simulink model "ventilator"  (R2020a)
settings: Solver=VariableStepAuto  StartTime=0.0  StopTime=20  FixedStep=0.001  MaxStep=0.01  RelTol=1e-3  AbsTol=1e-3
InitFcn:
  | load('params');
  | 
  | Transport_Delay = 0.001; % s
  | 
  | Zephyr_FS = 50; % SLPM
  | HSC_FS = 160; % mbar
  | 
  | P_supply =1; % bar
  | 
  | T_room = 20; % degC
  | RH_room = 0.1;
  | T_humidifier = 40; % degC
  | T_body = 37; % degC
  | 
  | L_tube = 1; % m
  | D_tube = 0.022; % m
  | L_trachea = 0.15; % m
  | D_trachea = 0.015; % m
  | 
  | Chamber_volume = 0.2; % L
  | FRC = 2; % L
  | 
  | % Conversion factors
  | cmH2O_to_Pa = 98.0665;
  | L_to_m3 = 1e-3;
undefined symbols (not defined in the file or in its folder): zephyr
libraries: fl_lib x101, nesl_utility x26
(part 2 of 2)

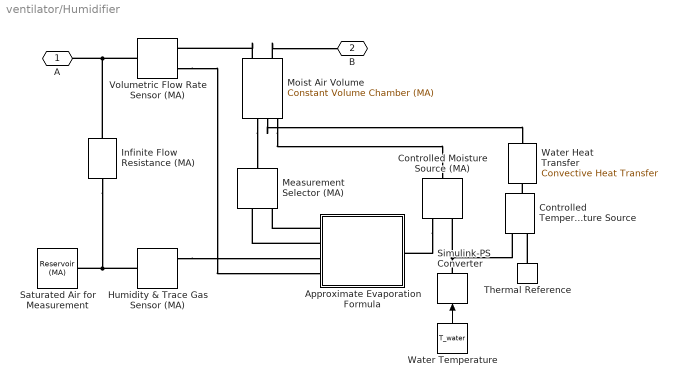
== system ventilator/Humidifier ==
  Approximate Evaporation Formula : Subsystem
  Controlled Temperature Source : fl_lib/Thermal/Thermal Sources/Controlled Temperature Source
      settings: SourceProductBaseCode=MT,SS
  Controlled Moisture Source (MA) : fl_lib/Moist Air/Sources/Moisture & Trace Gas Sources/Controlled Moisture Source (MA)  moisture_source_spec=foundation.enum.moisture_source_spec.vapor
      settings: SourceProductBaseCode=MT,SS  InternalSimscapePortConfiguration="{\"Bottom\":[],\"Left\":[{\"id\":\"S\",\"label\":\"S\",\"type\":\"foundation.moist_air.moist_air_source\"}],\"Right\":[{\"id\":\"M\",\"label\":\"M\",\"type\":\"input\"},{\"id\":\"T\",\"label\":\"T\",\"type\":\"input\"}],\"Top\":[]}"
  Humidity & Trace Gas Sensor (MA) : fl_lib/Moist Air/Sensors/Humidity & Trace Gas Sensor (MA)  moisture_spec=foundation.enum.moisture_spec.mole_fraction  trace_gas_spec=foundation.enum.trace_gas_spec.mass_fraction
      settings: SourceProductBaseCode=MT,SS  InternalSimscapePortConfiguration="{\"Bottom\":[],\"Left\":[{\"id\":\"A\",\"label\":\"A\",\"type\":\"foundation.moist_air.moist_air\"}],\"Right\":[{\"id\":\"W\",\"label\":\"W\",\"type\":\"output\"},{\"id\":\"G\",\"label\":\"G\",\"type\":\"output\"}],\"Top\":[]}"
  Infinite Flow Resistance (MA) : fl_lib/Moist Air/Elements/Infinite Flow Resistance (MA)  p_specify=off  p_priority=None  p=0 MPa  p_nominal_specify=off  p_nominal_unit=MPa  p_nominal_value=1  T_specify=off  T_priority=None  T=0 K  T_nominal_specify=off  T_nominal_unit=K  T_nominal_value=1  x_w_specify=off  x_w_priority=None  x_w=0  x_w_nominal_specify=off  x_w_nominal_unit=1  x_w_nominal_value=1  x_g_specify=off  x_g_priority=None  x_g=0  x_g_nominal_specify=off  x_g_nominal_unit=1  x_g_nominal_value=1
      settings: SourceProductBaseCode=MT,SS  InternalSimscapePortConfiguration="{\"Bottom\":[],\"Left\":[{\"id\":\"A\",\"label\":\"A\",\"type\":\"foundation.moist_air.moist_air\"}],\"Right\":[{\"id\":\"B\",\"label\":\"B\",\"type\":\"foundation.moist_air.moist_air\"}],\"Top\":[]}"
  Measurement Selector (MA) : fl_lib/Moist Air/Sensors/Measurement Selector (MA)  moisture_spec=foundation.enum.moisture_spec.mole_fraction  trace_gas_spec=foundation.enum.trace_gas_spec.mass_fraction
      settings: SourceProductBaseCode=MT,SS
  Moist Air Volume : fl_lib/Moist Air/Elements/Constant Volume Chamber (MA)  volume=V_humidifier m^3  num_ports=foundation.enum.num_ports.two  area_A=pi*D_tube^2/4 m^2  area_B=pi*D_tube^2/4 m^2  area_C=0.01 m^2  area_D=0.01 m^2  RH_ws=1  time_constant=1e-3 s  moisture_trace_gas_source=foundation.enum.moisture_trace_gas_source.controlled  moisture_source_spec=foundation.enum.moisture_source_spec.vapor  moisture_mass_flow=0 kg/s  moisture_temperature_spec=foundation.enum.temperature_spec.atmospheric  moisture_temperature=293.15 K  trace_gas_mass_flow=0 kg/s  trace_gas_temperature_spec=foundation.enum.temperature_spec.atmospheric  trace_gas_temperature=293.15 K  p_I_specify=off  p_I_priority=High  p_I=0.101325 MPa  p_I_nominal_specify=off  p_I_nominal_unit=MPa  p_I_nominal_value=1  T_I_specify=on  T_I_priority=High  T_I=T_room degC  T_I_nominal_specify=off  T_I_nominal_unit=K  T_I_nominal_value=1  RH_I_specify=on  RH_I_priority=High  RH_I=RH_room  RH_I_nominal_specify=off  RH_I_nominal_unit=1  RH_I_nominal_value=1  x_w_I_specify=off  x_w_I_priority=None  x_w_I=0  x_w_I_nominal_specify=off  x_w_I_nominal_unit=1  x_w_I_nominal_value=1  y_w_I_specify=off  y_w_I_priority=None  y_w_I=0  y_w_I_nominal_specify=off  y_w_I_nominal_unit=1  y_w_I_nominal_value=1  HR_I_specify=off  HR_I_priority=None  HR_I=0  HR_I_nominal_specify=off  HR_I_nominal_unit=1  HR_I_nominal_value=1  x_g_I_specify=off  x_g_I_priority=High  x_g_I=0  x_g_I_nominal_specify=off  x_g_I_nominal_unit=1  x_g_I_nominal_value=1  y_g_I_specify=off  y_g_I_priority=None  y_g_I=0  y_g_I_nominal_specify=off  y_g_I_nominal_unit=1  y_g_I_nominal_value=1
      settings: SourceProductBaseCode=MT,SS  InternalSimscapePortConfiguration="{\"Bottom\":[],\"Left\":[{\"id\":\"A\",\"label\":\"A\",\"type\":\"foundation.moist_air.moist_air\"},{\"id\":\"B\",\"label\":\"B\",\"type\":\"foundation.moist_air.moist_air\"}],\"Right\":[{\"id\":\"W\",\"label\":\"W\",\"type\":\"output\"},{\"id\":\"F\",\"label\":\"F\",\"type\":\"output\"},{\"id\":\"H\",\"label\":\"H\",\"type\":\"foundation.thermal.thermal\"},{\"id\":\"S\",\"label\":\"S\",\"type\":\"foundation.moist_air.moist_air_source\"}],\"Top\":[]}"
  Saturated Air for Measurement : fl_lib/Moist Air/Elements/Reservoir (MA)  pressure_spec=1  reservoir_pressure=0.101325 MPa  temperature_spec=2  reservoir_temperature=T_water degC  moisture_spec=1  reservoir_RH=1  reservoir_x_w=0.01  reservoir_y_w=0.01  reservoir_HR=0.01  trace_gas_spec=1  reservoir_x_g=0  reservoir_y_g=0.001  RH_ws=1  area_A=A_humidifier m^2
      settings: SourceProductBaseCode=MT,SS
  Simulink-PS Converter : nesl_utility/Simulink-PS Converter  PhysicalDomain=network_engine_domain  SubClassName=ps_input  LeftPortType=input  RightPortType=output  PseudoPeriodic=off  Frequencies=[]  NoiseDistribution=none  NoiseParameters=[]  Unit=degC  AffineConversion=on  FilteringAndDerivatives=provide  SimscapeFilterOrder=1  InputFilterTimeConstant=0.001  UdotUserProvided=0
      settings: SourceProductBaseCode=MT,SS
  Thermal Reference : fl_lib/Thermal/Thermal Elements/Thermal Reference
      settings: SourceProductBaseCode=MT,SS
  Volumetric Flow Rate Sensor (MA) : fl_lib/Moist Air/Sensors/Volumetric Flow Rate Sensor (MA)  volumetric_flow_conditions=foundation.enum.volumetric_flow_conditions.actual  p_std=0.101325 MPa  T_std=20 degC  RH_std=0.65
      settings: SourceProductBaseCode=MT,SS  InternalSimscapePortConfiguration="{\"Bottom\":[],\"Left\":[{\"id\":\"A\",\"label\":\"A\",\"type\":\"foundation.moist_air.moist_air\"}],\"Right\":[{\"id\":\"B\",\"label\":\"B\",\"type\":\"foundation.moist_air.moist_air\"},{\"id\":\"V\",\"label\":\"V\",\"type\":\"output\"}],\"Top\":[]}"
  Water Temperature : Constant  Value=T_water
  Water Heat Transfer : fl_lib/Thermal/Thermal Elements/Convective Heat Transfer  area=A_humidifier m^2  heat_tr_coeff=20 W/(m^2 * K)  T_specify=off  T_priority=None  T=0 K  T_nominal_specify=off  T_nominal_unit=K  T_nominal_value=1  Q_specify=off  Q_priority=None  Q=0 W  Q_nominal_specify=off  Q_nominal_unit=W  Q_nominal_value=1
      settings: SourceProductBaseCode=MT,SS
  A : PMIOPort  Side=Left
  B : PMIOPort  Port=2  Side=Right
  wires:
  Water Temperature/1 -> Simulink-PS Converter/1
  connections:
  Volumetric Flow Rate Sensor (MA)/LConn1 -- A/RConn1 -- Infinite Flow Resistance (MA)/RConn1
  Moist Air Volume/LConn1 -- Volumetric Flow Rate Sensor (MA)/RConn1
  Moist Air Volume/LConn2 -- B/RConn1
  Humidity & Trace Gas Sensor (MA)/RConn1 -- Approximate Evaporation Formula/LConn3
  Volumetric Flow Rate Sensor (MA)/RConn2 -- Approximate Evaporation Formula/LConn4
  Controlled Moisture Source (MA)/RConn1 -- Approximate Evaporation Formula/RConn1
  Moist Air Volume/RConn4 -- Controlled Moisture Source (MA)/LConn1
  Moist Air Volume/RConn2 -- Measurement Selector (MA)/LConn1
  Infinite Flow Resistance (MA)/LConn1 -- Saturated Air for Measurement/LConn1 -- Humidity & Trace Gas Sensor (MA)/LConn1
  Controlled Temperature Source/LConn1 -- Water Heat Transfer/RConn1
  Simulink-PS Converter/RConn1 -- Controlled Temperature Source/RConn1 -- Controlled Moisture Source (MA)/RConn2
  Moist Air Volume/RConn3 -- Water Heat Transfer/LConn1
  Thermal Reference/LConn1 -- Controlled Temperature Source/RConn2
  Approximate Evaporation Formula/LConn1 -- Measurement Selector (MA)/RConn1
  Approximate Evaporation Formula/LConn2 -- Measurement Selector (MA)/RConn3

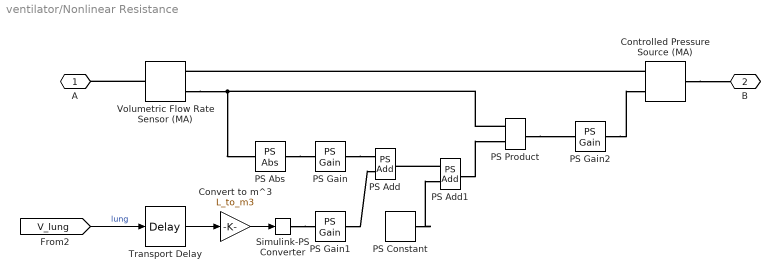
== system ventilator/Nonlinear Resistance ==
  Controlled Pressure Source (MA) : fl_lib/Moist Air/Sources/Controlled Pressure Source (MA)  power_spec=foundation.enum.power_spec.isentropic  area_A=pi*D_trachea^2/4 m^2  area_B=pi*D_trachea^2/4 m^2
      settings: SourceProductBaseCode=SS  InternalSimscapePortConfiguration="{\"Bottom\":[],\"Left\":[{\"id\":\"A\",\"label\":\"A\",\"type\":\"foundation.moist_air.moist_air\"},{\"id\":\"P\",\"label\":\"P\",\"type\":\"input\"}],\"Right\":[{\"id\":\"B\",\"label\":\"B\",\"type\":\"foundation.moist_air.moist_air\"}],\"Top\":[]}"
  Convert to m^3 : Gain  Gain=L_to_m3
  PS Abs : fl_lib/Physical Signals/Nonlinear Operators/PS Abs
      settings: SourceProductBaseCode=SS  InternalSimscapePortConfiguration="{\"Bottom\":[],\"Left\":[{\"id\":\"I\",\"label\":\"\",\"type\":\"input\"}],\"Right\":[{\"id\":\"O\",\"label\":\"\",\"type\":\"output\"}],\"Top\":[]}"
  PS Add : fl_lib/Physical Signals/Functions/PS Add
  PS Add1 : fl_lib/Physical Signals/Functions/PS Add
  PS Constant : fl_lib/Physical Signals/Sources/PS Constant  constant=R0 * 1e3 / 1e-3 Pa * s / m^3
  PS Gain : fl_lib/Physical Signals/Functions/PS Gain  gain=Kf * 1e3 / 1e-6 Pa * s^2 / m^6
  PS Gain1 : fl_lib/Physical Signals/Functions/PS Gain  gain=Kv * 1e3 / 1e-6 Pa * s / m^6
  PS Gain2 : fl_lib/Physical Signals/Functions/PS Gain  gain=-1
  PS Product : fl_lib/Physical Signals/Functions/PS Product
  Simulink-PS Converter : nesl_utility/Simulink-PS Converter  PhysicalDomain=network_engine_domain  SubClassName=ps_input  LeftPortType=input  RightPortType=output  PseudoPeriodic=off  Frequencies=[]  NoiseDistribution=none  NoiseParameters=[]  Unit=m^3  AffineConversion=off  FilteringAndDerivatives=provide  SimscapeFilterOrder=1  InputFilterTimeConstant=0.001  UdotUserProvided=0
  Transport Delay : TransportDelay  DelayTime=Transport_Delay  BufferSize=2048
  Volumetric Flow Rate Sensor (MA) : fl_lib/Moist Air/Sensors/Volumetric Flow Rate Sensor (MA)  volumetric_flow_conditions=foundation.enum.volumetric_flow_conditions.actual  p_std=0.101325 MPa  T_std=20 degC  RH_std=0.65
      settings: SourceProductBaseCode=SS  InternalSimscapePortConfiguration="{\"Bottom\":[],\"Left\":[{\"id\":\"A\",\"label\":\"A\",\"type\":\"foundation.moist_air.moist_air\"}],\"Right\":[{\"id\":\"B\",\"label\":\"B\",\"type\":\"foundation.moist_air.moist_air\"},{\"id\":\"V\",\"label\":\"V\",\"type\":\"output\"}],\"Top\":[]}"
  A : PMIOPort  Side=Left
  B : PMIOPort  Port=2  Side=Right
  wires:
  [V_lung] -> Transport Delay/1  "lung"
  Convert to m^3/1 -> Simulink-PS Converter/1
  Transport Delay/1 -> Convert to m^3/1
  connections:
  Volumetric Flow Rate Sensor (MA)/RConn2 -- PS Abs/LConn1 -- PS Product/LConn1
  Volumetric Flow Rate Sensor (MA)/LConn1 -- A/RConn1
  PS Abs/RConn1 -- PS Gain/LConn1
  PS Gain/RConn1 -- PS Add/LConn1
  PS Add1/LConn1 -- PS Add/RConn1
  PS Constant/RConn1 -- PS Add1/LConn2
  PS Add1/RConn1 -- PS Product/LConn2
  Simulink-PS Converter/RConn1 -- PS Gain1/LConn1
  PS Gain1/RConn1 -- PS Add/LConn2
  Controlled Pressure Source (MA)/LConn1 -- Volumetric Flow Rate Sensor (MA)/RConn1
  Controlled Pressure Source (MA)/RConn1 -- B/RConn1
  PS Gain2/RConn1 -- Controlled Pressure Source (MA)/LConn2
  PS Product/RConn1 -- PS Gain2/LConn1

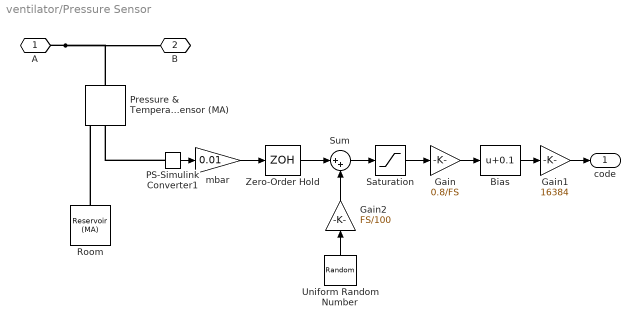
== system ventilator/Pressure Sensor ==
  Bias : Bias  Bias=0.1
  Gain : Gain  Gain=0.8/FS
  Gain1 : Gain  Gain=16384
  Gain2 : Gain  Gain=FS/100
  PS-Simulink Converter1 : nesl_utility/PS-Simulink Converter  PhysicalDomain=network_engine_domain  SubClassName=ps_output  LeftPortType=input  RightPortType=output  PseudoPeriodic=off  Frequencies=[]  Unit=inherit  AffineConversion=off
  Pressure & Temperature Sensor (MA) : fl_lib/Moist Air/Sensors/Pressure & Temperature Sensor (MA)
      settings: SourceProductBaseCode=MT,SS  InternalSimscapePortConfiguration="{\"Bottom\":[],\"Left\":[{\"id\":\"A\",\"label\":\"A\",\"type\":\"foundation.moist_air.moist_air\"}],\"Right\":[{\"id\":\"B\",\"label\":\"B\",\"type\":\"foundation.moist_air.moist_air\"},{\"id\":\"P\",\"label\":\"P\",\"type\":\"output\"},{\"id\":\"T\",\"label\":\"T\",\"type\":\"output\"}],\"Top\":[]}"
  Room : fl_lib/Moist Air/Elements/Reservoir (MA)  pressure_spec=foundation.enum.pressure_spec.atmospheric  reservoir_pressure=0.101325 MPa  temperature_spec=foundation.enum.temperature_spec.specified  reservoir_temperature=T_room degC  moisture_spec=foundation.enum.moisture_spec.relative_humidity  reservoir_RH=RH_room  reservoir_x_w=0.01  reservoir_y_w=0.01  reservoir_HR=0.01  trace_gas_spec=foundation.enum.trace_gas_spec.mass_fraction  reservoir_x_g=0  reservoir_y_g=0.001  RH_ws=1  area_A=pi*D_tube^2/4 m^2
      settings: SourceProductBaseCode=MT,SS
  Saturation : Saturate  UpperLimit=FS  LowerLimit=0
  Sum : Sum  Inputs=|++
  Uniform Random Number : UniformRandomNumber  SampleTime=Ts
  Zero-Order Hold : ZeroOrderHold  SampleTime=Ts
  mbar : Gain  Gain=0.01
  A : PMIOPort  Side=Left
  B : PMIOPort  Port=2  Side=Right
  code : Outport
  wires:
  Saturation/1 -> Gain/1
  Gain1/1 -> code/1
  Bias/1 -> Gain1/1
  Gain/1 -> Bias/1
  Sum/1 -> Saturation/1
  mbar/1 -> Zero-Order Hold/1
  Zero-Order Hold/1 -> Sum/1
  Uniform Random Number/1 -> Gain2/1
  Gain2/1 -> Sum/2
  PS-Simulink Converter1/1 -> mbar/1
  connections:
  PS-Simulink Converter1/LConn1 -- Pressure & Temperature Sensor (MA)/RConn2
  Room/LConn1 -- Pressure & Temperature Sensor (MA)/RConn1
  A/RConn1 -- B/RConn1 -- Pressure & Temperature Sensor (MA)/LConn1

== system ventilator/Proportional Inlet Valve ==
  duty_cycle : Inport
  Apply Actual Conditions : Subsystem
  Controlled Volumetric Flow Rate Source (MA) : fl_lib/Moist Air/Sources/Controlled Volumetric Flow Rate Source (MA)  power_spec=foundation.enum.power_spec.isentropic  volumetric_flow_conditions=foundation.enum.volumetric_flow_conditions.actual  p_std=0.101325 MPa  T_std=20 degC  RH_std=0.65  area_A=pi*D_tube^2/4 m^2  area_B=pi*D_tube^2/4 m^2
      settings: SourceProductBaseCode=SS  InternalSimscapePortConfiguration="{\"Bottom\":[],\"Left\":[{\"id\":\"A\",\"label\":\"A\",\"type\":\"foundation.moist_air.moist_air\"},{\"id\":\"V\",\"label\":\"V\",\"type\":\"input\"}],\"Right\":[{\"id\":\"B\",\"label\":\"B\",\"type\":\"foundation.moist_air.moist_air\"}],\"Top\":[]}"
  PS Constant : fl_lib/Physical Signals/Sources/PS Constant  constant=1e5 * valve.preload_offset Pa
  PS Lookup Table (2D) : fl_lib/Physical Signals/Lookup Tables/PS Lookup Table (2D)  x1=1e5 * valve.pressure Pa  x2=valve.duty_cycle  f=(1e-3/60) * valve.flow_rate m^3/s  interp_method=simscape.enum.interpolation.linear  extrap_method=simscape.enum.extrapolation.linear
      settings: SourceProductBaseCode=SS
  PS Subtract : fl_lib/Physical Signals/Functions/PS Subtract
  PS Transfer Function : fl_lib/Physical Signals/Linear Operators/PS Transfer Function  transfer_function_type=foundation.enum.transfer_function_type.lag  T=tau s  T1=2 s  T2=1 s  y0=0 m^3/s
      settings: SourceProductBaseCode=SS  InternalSimscapePortConfiguration="{\"Bottom\":[],\"Left\":[{\"id\":\"U\",\"label\":\"\",\"type\":\"input\"}],\"Right\":[{\"id\":\"Y\",\"label\":\"\",\"type\":\"output\"}],\"Top\":[]}"
  Pressure & Temperature Sensor (MA) : fl_lib/Moist Air/Sensors/Pressure & Temperature Sensor (MA)
      settings: SourceProductBaseCode=MT,SS  InternalSimscapePortConfiguration="{\"Bottom\":[],\"Left\":[{\"id\":\"A\",\"label\":\"A\",\"type\":\"foundation.moist_air.moist_air\"}],\"Right\":[{\"id\":\"B\",\"label\":\"B\",\"type\":\"foundation.moist_air.moist_air\"},{\"id\":\"P\",\"label\":\"P\",\"type\":\"output\"},{\"id\":\"T\",\"label\":\"T\",\"type\":\"output\"}],\"Top\":[]}"
  Saturation : Saturate  UpperLimit=100  LowerLimit=0
  Simulink-PS Converter : nesl_utility/Simulink-PS Converter  PhysicalDomain=network_engine_domain  SubClassName=ps_input  LeftPortType=input  RightPortType=output  PseudoPeriodic=off  Frequencies=[]  NoiseDistribution=none  NoiseParameters=[]  Unit=1  AffineConversion=off  FilteringAndDerivatives=provide  SimscapeFilterOrder=1  InputFilterTimeConstant=0.001  UdotUserProvided=0
  A : PMIOPort  Side=Left
  B : PMIOPort  Port=2  Side=Right
  wires:
  duty_cycle/1 -> Saturation/1
  Saturation/1 -> Simulink-PS Converter/1
  connections:
  Controlled Volumetric Flow Rate Source (MA)/LConn1 -- Pressure & Temperature Sensor (MA)/LConn1 -- A/RConn1
  Controlled Volumetric Flow Rate Source (MA)/RConn1 -- Pressure & Temperature Sensor (MA)/RConn1 -- B/RConn1
  PS Lookup Table (2D)/RConn1 -- Apply Actual Conditions/LConn1
  PS Transfer Function/RConn1 -- Controlled Volumetric Flow Rate Source (MA)/LConn2
  Apply Actual Conditions/RConn1 -- PS Transfer Function/LConn1
  PS Lookup Table (2D)/LConn2 -- Simulink-PS Converter/RConn1
  PS Subtract/LConn1 -- Pressure & Temperature Sensor (MA)/RConn2
  PS Subtract/RConn1 -- PS Lookup Table (2D)/LConn1
  PS Subtract/LConn2 -- PS Constant/RConn1

== system ventilator/Safety Vent Trap ==
  PS Transfer Function : fl_lib/Physical Signals/Linear Operators/PS Transfer Function  transfer_function_type=foundation.enum.transfer_function_type.lag  T=tau s  T1=2 s  T2=1 s  y0=1e-10 m^2
      settings: SourceProductBaseCode=SS  InternalSimscapePortConfiguration="{\"Bottom\":[],\"Left\":[{\"id\":\"U\",\"label\":\"\",\"type\":\"input\"}],\"Right\":[{\"id\":\"Y\",\"label\":\"\",\"type\":\"output\"}],\"Top\":[]}"
  Pressure & Temperature Sensor (MA) : fl_lib/Moist Air/Sensors/Pressure & Temperature Sensor (MA)
      settings: SourceProductBaseCode=MT,SS  InternalSimscapePortConfiguration="{\"Bottom\":[],\"Left\":[{\"id\":\"A\",\"label\":\"A\",\"type\":\"foundation.moist_air.moist_air\"}],\"Right\":[{\"id\":\"B\",\"label\":\"B\",\"type\":\"foundation.moist_air.moist_air\"},{\"id\":\"P\",\"label\":\"P\",\"type\":\"output\"},{\"id\":\"T\",\"label\":\"T\",\"type\":\"output\"}],\"Top\":[]}"
  Pressure to Area : fl_lib/Physical Signals/Lookup Tables/PS Lookup Table (1D)  x=[-0.2 -0.1 0 0.2 0.5 0.8 1 1.1 1.2]*(p_max - p_crack) + p_crack Pa  f=[0 0 0 0.2 0.5 0.8 1 1 1]*(pi*D_nozzle^2/4 - 1e-10) + 1e-10 m^2  interp_method=simscape.enum.interpolation.smooth  extrap_method=simscape.enum.extrapolation.nearest
      settings: SourceProductBaseCode=MT,SS
  Valve : fl_lib/Moist Air/Elements/Local Restriction (MA)  restriction_type=foundation.enum.restriction_type.variable  restriction_area=0.001 m^2  min_area=1e-10 m^2  max_area=pi*D_nozzle^2/4 m^2  area=pi*D_tube^2/4 m^2  Cd=0.8  B_lam=0.999
      settings: SourceProductBaseCode=MT,SS
  A : PMIOPort  Side=Left
  B : PMIOPort  Port=2  Side=Right
  connections:
  Pressure & Temperature Sensor (MA)/LConn1 -- Valve/LConn1 -- A/RConn1
  Pressure & Temperature Sensor (MA)/RConn1 -- Valve/RConn1 -- B/RConn1
  Pressure & Temperature Sensor (MA)/RConn2 -- Pressure to Area/LConn1
  PS Transfer Function/LConn1 -- Pressure to Area/RConn1
  PS Transfer Function/RConn1 -- Valve/LConn2

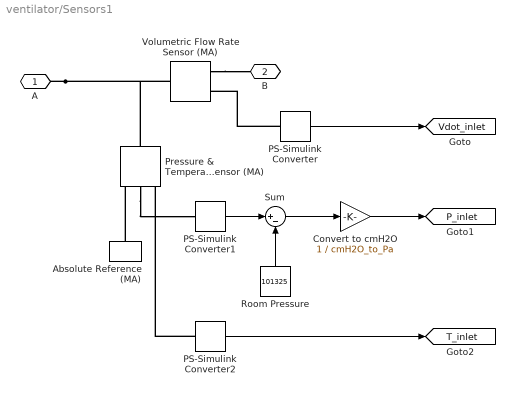
== system ventilator/Sensors1 ==
  Absolute Reference (MA) : fl_lib/Moist Air/Elements/Absolute Reference (MA)
      settings: SourceProductBaseCode=MT,SS
  Convert to cmH2O : Gain  Gain=1 / cmH2O_to_Pa
  PS-Simulink Converter : nesl_utility/PS-Simulink Converter  PhysicalDomain=network_engine_domain  SubClassName=ps_output  LeftPortType=input  RightPortType=output  PseudoPeriodic=off  Frequencies=[]  Unit=l/min  AffineConversion=off
      settings: SourceProductBaseCode=MT,SS
  PS-Simulink Converter1 : nesl_utility/PS-Simulink Converter  PhysicalDomain=network_engine_domain  SubClassName=ps_output  LeftPortType=input  RightPortType=output  PseudoPeriodic=off  Frequencies=[]  Unit=Pa  AffineConversion=off
      settings: SourceProductBaseCode=MT,SS
  PS-Simulink Converter2 : nesl_utility/PS-Simulink Converter  PhysicalDomain=network_engine_domain  SubClassName=ps_output  LeftPortType=input  RightPortType=output  PseudoPeriodic=off  Frequencies=[]  Unit=K  AffineConversion=off
      settings: SourceProductBaseCode=MT,SS
  Pressure & Temperature Sensor (MA) : fl_lib/Moist Air/Sensors/Pressure & Temperature Sensor (MA)
      settings: SourceProductBaseCode=MT,SS  InternalSimscapePortConfiguration="{\"Bottom\":[],\"Left\":[{\"id\":\"A\",\"label\":\"A\",\"type\":\"foundation.moist_air.moist_air\"}],\"Right\":[{\"id\":\"B\",\"label\":\"B\",\"type\":\"foundation.moist_air.moist_air\"},{\"id\":\"P\",\"label\":\"P\",\"type\":\"output\"},{\"id\":\"T\",\"label\":\"T\",\"type\":\"output\"}],\"Top\":[]}"
  Room Pressure : Constant  Value=101325
  Sum : Sum  Inputs=|+-
  Volumetric Flow Rate Sensor (MA) : fl_lib/Moist Air/Sensors/Volumetric Flow Rate Sensor (MA)  volumetric_flow_conditions=foundation.enum.volumetric_flow_conditions.actual  p_std=0.101325 MPa  T_std=20 degC  RH_std=0.65
      settings: SourceProductBaseCode=MT,SS  InternalSimscapePortConfiguration="{\"Bottom\":[],\"Left\":[{\"id\":\"A\",\"label\":\"A\",\"type\":\"foundation.moist_air.moist_air\"}],\"Right\":[{\"id\":\"B\",\"label\":\"B\",\"type\":\"foundation.moist_air.moist_air\"},{\"id\":\"V\",\"label\":\"V\",\"type\":\"output\"}],\"Top\":[]}"
  A : PMIOPort  Side=Left
  B : PMIOPort  Port=2  Side=Right
  tag scope: P_inlet=global, T_inlet=global, Vdot_inlet=global
  wires:
  Room Pressure/1 -> Sum/2
  Sum/1 -> Convert to cmH2O/1
  PS-Simulink Converter1/1 -> Sum/1
  Convert to cmH2O/1 -> [P_inlet]
  PS-Simulink Converter/1 -> [Vdot_inlet]
  PS-Simulink Converter2/1 -> [T_inlet]
  connections:
  Pressure & Temperature Sensor (MA)/RConn2 -- PS-Simulink Converter1/LConn1
  Absolute Reference (MA)/LConn1 -- Pressure & Temperature Sensor (MA)/RConn1
  Volumetric Flow Rate Sensor (MA)/RConn1 -- B/RConn1
  A/RConn1 -- Pressure & Temperature Sensor (MA)/LConn1 -- Volumetric Flow Rate Sensor (MA)/LConn1
  PS-Simulink Converter/LConn1 -- Volumetric Flow Rate Sensor (MA)/RConn2
  PS-Simulink Converter2/LConn1 -- Pressure & Temperature Sensor (MA)/RConn3

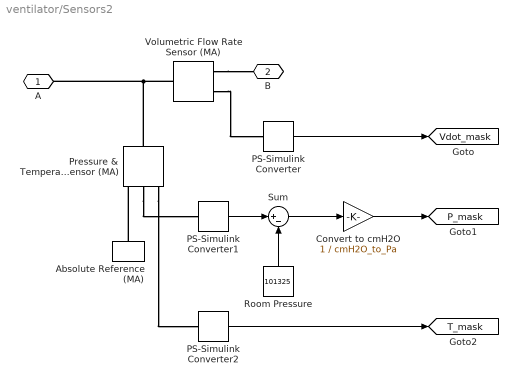
== system ventilator/Sensors2 ==
  Absolute Reference (MA) : fl_lib/Moist Air/Elements/Absolute Reference (MA)
      settings: SourceProductBaseCode=MT,SS
  Convert to cmH2O : Gain  Gain=1 / cmH2O_to_Pa
  PS-Simulink Converter : nesl_utility/PS-Simulink Converter  PhysicalDomain=network_engine_domain  SubClassName=ps_output  LeftPortType=input  RightPortType=output  PseudoPeriodic=off  Frequencies=[]  Unit=l/min  AffineConversion=off
      settings: SourceProductBaseCode=MT,SS
  PS-Simulink Converter1 : nesl_utility/PS-Simulink Converter  PhysicalDomain=network_engine_domain  SubClassName=ps_output  LeftPortType=input  RightPortType=output  PseudoPeriodic=off  Frequencies=[]  Unit=Pa  AffineConversion=off
      settings: SourceProductBaseCode=MT,SS
  PS-Simulink Converter2 : nesl_utility/PS-Simulink Converter  PhysicalDomain=network_engine_domain  SubClassName=ps_output  LeftPortType=input  RightPortType=output  PseudoPeriodic=off  Frequencies=[]  Unit=K  AffineConversion=off
      settings: SourceProductBaseCode=MT,SS
  Pressure & Temperature Sensor (MA) : fl_lib/Moist Air/Sensors/Pressure & Temperature Sensor (MA)
      settings: SourceProductBaseCode=MT,SS  InternalSimscapePortConfiguration="{\"Bottom\":[],\"Left\":[{\"id\":\"A\",\"label\":\"A\",\"type\":\"foundation.moist_air.moist_air\"}],\"Right\":[{\"id\":\"B\",\"label\":\"B\",\"type\":\"foundation.moist_air.moist_air\"},{\"id\":\"P\",\"label\":\"P\",\"type\":\"output\"},{\"id\":\"T\",\"label\":\"T\",\"type\":\"output\"}],\"Top\":[]}"
  Room Pressure : Constant  Value=101325
  Sum : Sum  Inputs=|+-
  Volumetric Flow Rate Sensor (MA) : fl_lib/Moist Air/Sensors/Volumetric Flow Rate Sensor (MA)  volumetric_flow_conditions=foundation.enum.volumetric_flow_conditions.actual  p_std=0.101325 MPa  T_std=20 degC  RH_std=0.65
      settings: SourceProductBaseCode=MT,SS  InternalSimscapePortConfiguration="{\"Bottom\":[],\"Left\":[{\"id\":\"A\",\"label\":\"A\",\"type\":\"foundation.moist_air.moist_air\"}],\"Right\":[{\"id\":\"B\",\"label\":\"B\",\"type\":\"foundation.moist_air.moist_air\"},{\"id\":\"V\",\"label\":\"V\",\"type\":\"output\"}],\"Top\":[]}"
  A : PMIOPort  Side=Left
  B : PMIOPort  Port=2  Side=Right
  tag scope: P_mask=global, T_mask=global, Vdot_mask=global
  wires:
  PS-Simulink Converter/1 -> [Vdot_mask]
  Convert to cmH2O/1 -> [P_mask]
  PS-Simulink Converter1/1 -> Sum/1
  Sum/1 -> Convert to cmH2O/1
  Room Pressure/1 -> Sum/2
  PS-Simulink Converter2/1 -> [T_mask]
  connections:
  Volumetric Flow Rate Sensor (MA)/LConn1 -- Pressure & Temperature Sensor (MA)/LConn1 -- A/RConn1
  Volumetric Flow Rate Sensor (MA)/RConn1 -- B/RConn1
  Volumetric Flow Rate Sensor (MA)/RConn2 -- PS-Simulink Converter/LConn1
  Absolute Reference (MA)/LConn1 -- Pressure & Temperature Sensor (MA)/RConn1
  Pressure & Temperature Sensor (MA)/RConn2 -- PS-Simulink Converter1/LConn1
  Pressure & Temperature Sensor (MA)/RConn3 -- PS-Simulink Converter2/LConn1

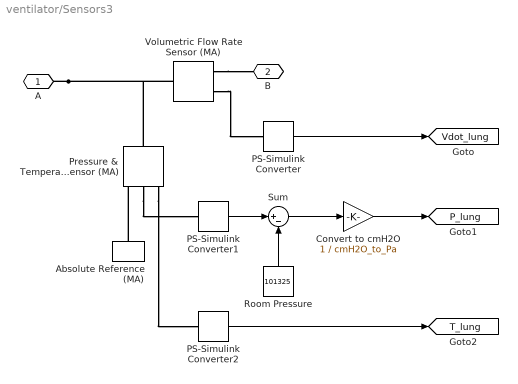
== system ventilator/Sensors3 ==
  Absolute Reference (MA) : fl_lib/Moist Air/Elements/Absolute Reference (MA)
      settings: SourceProductBaseCode=MT,SS
  Convert to cmH2O : Gain  Gain=1 / cmH2O_to_Pa
  PS-Simulink Converter : nesl_utility/PS-Simulink Converter  PhysicalDomain=network_engine_domain  SubClassName=ps_output  LeftPortType=input  RightPortType=output  PseudoPeriodic=off  Frequencies=[]  Unit=l/min  AffineConversion=off
      settings: SourceProductBaseCode=MT,SS
  PS-Simulink Converter1 : nesl_utility/PS-Simulink Converter  PhysicalDomain=network_engine_domain  SubClassName=ps_output  LeftPortType=input  RightPortType=output  PseudoPeriodic=off  Frequencies=[]  Unit=Pa  AffineConversion=off
      settings: SourceProductBaseCode=MT,SS
  PS-Simulink Converter2 : nesl_utility/PS-Simulink Converter  PhysicalDomain=network_engine_domain  SubClassName=ps_output  LeftPortType=input  RightPortType=output  PseudoPeriodic=off  Frequencies=[]  Unit=K  AffineConversion=off
      settings: SourceProductBaseCode=MT,SS
  Pressure & Temperature Sensor (MA) : fl_lib/Moist Air/Sensors/Pressure & Temperature Sensor (MA)
      settings: SourceProductBaseCode=MT,SS  InternalSimscapePortConfiguration="{\"Bottom\":[],\"Left\":[{\"id\":\"A\",\"label\":\"A\",\"type\":\"foundation.moist_air.moist_air\"}],\"Right\":[{\"id\":\"B\",\"label\":\"B\",\"type\":\"foundation.moist_air.moist_air\"},{\"id\":\"P\",\"label\":\"P\",\"type\":\"output\"},{\"id\":\"T\",\"label\":\"T\",\"type\":\"output\"}],\"Top\":[]}"
  Room Pressure : Constant  Value=101325
  Sum : Sum  Inputs=|+-
  Volumetric Flow Rate Sensor (MA) : fl_lib/Moist Air/Sensors/Volumetric Flow Rate Sensor (MA)  volumetric_flow_conditions=foundation.enum.volumetric_flow_conditions.actual  p_std=0.101325 MPa  T_std=20 degC  RH_std=0.65
      settings: SourceProductBaseCode=MT,SS  InternalSimscapePortConfiguration="{\"Bottom\":[],\"Left\":[{\"id\":\"A\",\"label\":\"A\",\"type\":\"foundation.moist_air.moist_air\"}],\"Right\":[{\"id\":\"B\",\"label\":\"B\",\"type\":\"foundation.moist_air.moist_air\"},{\"id\":\"V\",\"label\":\"V\",\"type\":\"output\"}],\"Top\":[]}"
  A : PMIOPort  Side=Left
  B : PMIOPort  Port=2  Side=Right
  tag scope: P_lung=global, T_lung=global, Vdot_lung=global
  wires:
  Room Pressure/1 -> Sum/2
  Sum/1 -> Convert to cmH2O/1
  PS-Simulink Converter1/1 -> Sum/1
  Convert to cmH2O/1 -> [P_lung]
  PS-Simulink Converter/1 -> [Vdot_lung]
  PS-Simulink Converter2/1 -> [T_lung]
  connections:
  Pressure & Temperature Sensor (MA)/RConn2 -- PS-Simulink Converter1/LConn1
  Absolute Reference (MA)/LConn1 -- Pressure & Temperature Sensor (MA)/RConn1
  Volumetric Flow Rate Sensor (MA)/RConn2 -- PS-Simulink Converter/LConn1
  Volumetric Flow Rate Sensor (MA)/RConn1 -- B/RConn1
  A/RConn1 -- Pressure & Temperature Sensor (MA)/LConn1 -- Volumetric Flow Rate Sensor (MA)/LConn1
  Pressure & Temperature Sensor (MA)/RConn3 -- PS-Simulink Converter2/LConn1

== system ventilator/Sensors4 ==
  Absolute Reference (MA) : fl_lib/Moist Air/Elements/Absolute Reference (MA)
      settings: SourceProductBaseCode=MT,SS
  Convert to cmH2O : Gain  Gain=1 / cmH2O_to_Pa
  PS-Simulink Converter : nesl_utility/PS-Simulink Converter  PhysicalDomain=network_engine_domain  SubClassName=ps_output  LeftPortType=input  RightPortType=output  PseudoPeriodic=off  Frequencies=[]  Unit=l/min  AffineConversion=off
      settings: SourceProductBaseCode=MT,SS
  PS-Simulink Converter1 : nesl_utility/PS-Simulink Converter  PhysicalDomain=network_engine_domain  SubClassName=ps_output  LeftPortType=input  RightPortType=output  PseudoPeriodic=off  Frequencies=[]  Unit=Pa  AffineConversion=off
      settings: SourceProductBaseCode=MT,SS
  PS-Simulink Converter2 : nesl_utility/PS-Simulink Converter  PhysicalDomain=network_engine_domain  SubClassName=ps_output  LeftPortType=input  RightPortType=output  PseudoPeriodic=off  Frequencies=[]  Unit=K  AffineConversion=off
      settings: SourceProductBaseCode=MT,SS
  Pressure & Temperature Sensor (MA) : fl_lib/Moist Air/Sensors/Pressure & Temperature Sensor (MA)
      settings: SourceProductBaseCode=MT,SS  InternalSimscapePortConfiguration="{\"Bottom\":[],\"Left\":[{\"id\":\"A\",\"label\":\"A\",\"type\":\"foundation.moist_air.moist_air\"}],\"Right\":[{\"id\":\"B\",\"label\":\"B\",\"type\":\"foundation.moist_air.moist_air\"},{\"id\":\"P\",\"label\":\"P\",\"type\":\"output\"},{\"id\":\"T\",\"label\":\"T\",\"type\":\"output\"}],\"Top\":[]}"
  Room Pressure : Constant  Value=101325
  Sum : Sum  Inputs=|+-
  Volumetric Flow Rate Sensor (MA) : fl_lib/Moist Air/Sensors/Volumetric Flow Rate Sensor (MA)  volumetric_flow_conditions=foundation.enum.volumetric_flow_conditions.actual  p_std=0.101325 MPa  T_std=20 degC  RH_std=0.65
      settings: SourceProductBaseCode=MT,SS  InternalSimscapePortConfiguration="{\"Bottom\":[],\"Left\":[{\"id\":\"A\",\"label\":\"A\",\"type\":\"foundation.moist_air.moist_air\"}],\"Right\":[{\"id\":\"B\",\"label\":\"B\",\"type\":\"foundation.moist_air.moist_air\"},{\"id\":\"V\",\"label\":\"V\",\"type\":\"output\"}],\"Top\":[]}"
  A : PMIOPort  Side=Left
  B : PMIOPort  Port=2  Side=Right
  tag scope: P_trap=global, T_trap=global, Vdot_trap=global
  wires:
  PS-Simulink Converter2/1 -> [T_trap]
  PS-Simulink Converter/1 -> [Vdot_trap]
  Convert to cmH2O/1 -> [P_trap]
  PS-Simulink Converter1/1 -> Sum/1
  Sum/1 -> Convert to cmH2O/1
  Room Pressure/1 -> Sum/2
  connections:
  Pressure & Temperature Sensor (MA)/RConn3 -- PS-Simulink Converter2/LConn1
  Volumetric Flow Rate Sensor (MA)/LConn1 -- Pressure & Temperature Sensor (MA)/LConn1 -- A/RConn1
  Volumetric Flow Rate Sensor (MA)/RConn1 -- B/RConn1
  Volumetric Flow Rate Sensor (MA)/RConn2 -- PS-Simulink Converter/LConn1
  Absolute Reference (MA)/LConn1 -- Pressure & Temperature Sensor (MA)/RConn1
  Pressure & Temperature Sensor (MA)/RConn2 -- PS-Simulink Converter1/LConn1

== system ventilator/Volume Data ==
  Constant : Constant  Value=FRC
  Convert to L : Gain  Gain=1/(L_to_m3)
  Ideal Translational Motion Sensor : fl_lib/Mechanical/Mechanical Sensors/Ideal Translational Motion Sensor  offset=FRC * L_to_m3 m
      settings: SourceProductBaseCode=MT,SS
  PS-Simulink Converter : nesl_utility/PS-Simulink Converter  PhysicalDomain=network_engine_domain  SubClassName=ps_output  LeftPortType=input  RightPortType=output  PseudoPeriodic=off  Frequencies=[]  Unit=m  AffineConversion=off
      settings: SourceProductBaseCode=MT,SS
  Sum : Sum  Inputs=|+-
  R : PMIOPort  Side=Left
  C : PMIOPort  Port=2  Side=Right
  tag scope: V_lung=global
  wires:
  PS-Simulink Converter/1 -> Convert to L/1
  Constant/1 -> Sum/2
  Convert to L/1 -> Sum/1
  Sum/1 -> [V_lung]
  connections:
  Ideal Translational Motion Sensor/LConn1 -- R/RConn1
  Ideal Translational Motion Sensor/RConn1 -- C/RConn1
  Ideal Translational Motion Sensor/RConn3 -- PS-Simulink Converter/LConn1

== system ventilator/lungs ssc vs. sim ==
  Mux1 : Mux  Inputs=2
  Mux2 : Mux  Inputs=2
  Scope : Scope  NumInputPorts=2
  human lung : Subsystem  mask(Human Lung){E=2.37, R0=0.47, Kv=-0.45, Kf=0.01, K1=0.83, tau1=0.01, tau2=3.89, Ts=0.01, N=32, d=0.01}
      mask prompts: E "E (total lung elasticity) [kPa/l]"; R0 "R0 (airways static resistance) [kPas/l]"; Kv "Kv (volume resistance coefficient) [kPas/l^2]"; Kf "Kf (flow resistance coefficient) [kPas^2/l^2]"; K1 "K1 (viscosity ratio) [−]"; tau1 "tau1 (lung elasticity time constant) [s]"; tau2 "tau2 (lung viscosity time constant) [s]"; Ts "Sample time [s]"; N "Max buffer length"; d "Max deviation threshold"
      mask help: Human Lung
      mask DialogControl Container2 Prompt: Lung Parameters
      mask DialogControl Container3 Prompt: Derivative computation
      mask DialogControl AlgoName Prompt: Adaptive Windows Polynomial Least-Squares Estimator
      mask DialogControl AlgoDescription Prompt: The parameter N identifies the maximum window length for buffering the data. Therefore, the window on which the least-squares algorithm operates on will automatically adapts its length from a minimum of 2 to a maximum of N samples. The greater is N, the more filtered is the derivative. The parameter d allows specifying the maximum deviation threshold for the algorithm. During the validation phase, indeed, the window's length is considered valid if all the computed values from the linear regressor lie within this threshold wrt their corresponding sample values. If not, the window's length is reduced by one step. At each instance, a trial on a window's length enlarged by one step is performed. Therefore, iteration by iteration, the window's length can be adapted by only one step change.
      mask Display: image('../assets/lung.png');
  wires:
  [P_mask] -> human lung/1(Pm)  "mask"
  human lung/2(V) -> Mux2/2  "sim"
  Mux1/1 -> Scope/1
  human lung/1(Vdot) -> Mux1/2  "sim"
  [Vdot_lung] -> Mux1/1  "ssc"
  [V_lung] -> Mux2/1  "ssc"
  Mux2/1 -> Scope/2

== system ventilator/CFB Outlet Valve/Apply Actual Conditions ==
  Qi : Inport
  To : Inport  Port=2
  Po : Inport  Port=3
  Constant : Constant  Value=273.15+20
  Constant1 : Constant  Value=101325
  Convert to Pa : Gain  Gain=1e5
  Divide : Product  Inputs=*/
  Divide1 : Product  Inputs=*/
  Product : Product
  Product1 : Product
  Qo : Outport
  wires:
  Qi/1 -> Product/1
  Product/1 -> Product1/1
  Product1/1 -> Qo/1
  Divide/1 -> Product/2
  Divide1/1 -> Product1/2
  Constant/1 -> Divide/1
  Constant1/1 -> Divide1/1
  To/1 -> Divide/2
  Convert to Pa/1 -> Divide1/2
  Po/1 -> Convert to Pa/1

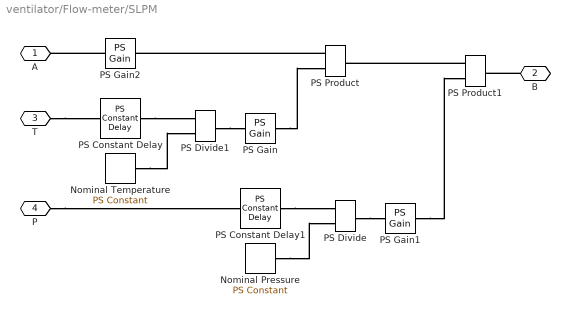
== system ventilator/Flow-meter/SLPM ==
  Nominal Pressure : fl_lib/Physical Signals/Sources/PS Constant  constant=101325 Pa
  Nominal Temperature : fl_lib/Physical Signals/Sources/PS Constant  constant=273.15+20 K
  PS Constant Delay : fl_lib/Physical Signals/Delays/PS Constant Delay  InputHistory=273.15+T_room K  DelayTime=Transport_Delay s
      settings: SourceProductBaseCode=SS  InternalSimscapePortConfiguration="{\"Bottom\":[],\"Left\":[{\"id\":\"U\",\"label\":\"U\",\"type\":\"input\"}],\"Right\":[{\"id\":\"Y\",\"label\":\"Y\",\"type\":\"output\"}],\"Top\":[]}"
  PS Constant Delay1 : fl_lib/Physical Signals/Delays/PS Constant Delay  InputHistory=101325 Pa  DelayTime=Transport_Delay s
      settings: SourceProductBaseCode=SS  InternalSimscapePortConfiguration="{\"Bottom\":[],\"Left\":[{\"id\":\"U\",\"label\":\"U\",\"type\":\"input\"}],\"Right\":[{\"id\":\"Y\",\"label\":\"Y\",\"type\":\"output\"}],\"Top\":[]}"
  PS Divide : fl_lib/Physical Signals/Functions/PS Divide
      settings: SourceProductBaseCode=SS
  PS Divide1 : fl_lib/Physical Signals/Functions/PS Divide
      settings: SourceProductBaseCode=SS
  PS Gain : fl_lib/Physical Signals/Functions/PS Gain  gain=273.15/293.15
  PS Gain1 : fl_lib/Physical Signals/Functions/PS Gain  gain=14.696/14.504
  PS Gain2 : fl_lib/Physical Signals/Functions/PS Gain  gain=1e3/(1/60)
  PS Product : fl_lib/Physical Signals/Functions/PS Product
  PS Product1 : fl_lib/Physical Signals/Functions/PS Product
  A : PMIOPort  Side=Left
  B : PMIOPort  Port=2  Side=Right
  T : PMIOPort  Port=3  Side=Left
  P : PMIOPort  Port=4  Side=Left
  connections:
  PS Product/LConn1 -- PS Gain2/RConn1
  PS Product1/LConn1 -- PS Product/RConn1
  B/RConn1 -- PS Product1/RConn1
  PS Gain/RConn1 -- PS Product/LConn2
  PS Gain1/RConn1 -- PS Product1/LConn2
  T/RConn1 -- PS Constant Delay/LConn1
  P/RConn1 -- PS Constant Delay1/LConn1
  PS Constant Delay1/RConn1 -- PS Divide/LConn1
  Nominal Pressure/RConn1 -- PS Divide/LConn2
  PS Constant Delay/RConn1 -- PS Divide1/LConn1
  Nominal Temperature/RConn1 -- PS Divide1/LConn2
  PS Divide1/RConn1 -- PS Gain/LConn1
  PS Divide/RConn1 -- PS Gain1/LConn1
  PS Gain2/LConn1 -- A/RConn1

== system ventilator/Humidifier/Approximate Evaporation Formula ==
  Empirical Factor : fl_lib/Physical Signals/Functions/PS Gain  gain=5e-8 kg/J
      settings: SourceProductBaseCode=MT,SS
  Flow Area : fl_lib/Physical Signals/Functions/PS Gain  gain=1 / (pi*D_tube^2/4) 1/m^2
      settings: SourceProductBaseCode=MT,SS
  PS Product : fl_lib/Physical Signals/Functions/PS Product
      settings: SourceProductBaseCode=MT,SS
  PS Product1 : fl_lib/Physical Signals/Functions/PS Product
      settings: SourceProductBaseCode=MT,SS
  PS Subtract : fl_lib/Physical Signals/Functions/PS Subtract
      settings: SourceProductBaseCode=MT,SS
  Water Surface Area : fl_lib/Physical Signals/Functions/PS Gain  gain=A_humidifier m^2
      settings: SourceProductBaseCode=MT,SS
  p : PMIOPort  Side=Left
  y_w : PMIOPort  Port=2  Side=Left
  y_ws : PMIOPort  Port=3  Side=Left
  Vdot : PMIOPort  Port=4  Side=Left
  mdot_w : PMIOPort  Port=5  Side=Right
  connections:
  y_w/RConn1 -- PS Subtract/LConn2
  y_ws/RConn1 -- PS Subtract/LConn1
  p/RConn1 -- PS Product/LConn1
  PS Product/LConn2 -- PS Subtract/RConn1
  PS Product/RConn1 -- PS Product1/LConn1
  Flow Area/RConn1 -- PS Product1/LConn2
  Empirical Factor/LConn1 -- PS Product1/RConn1
  Water Surface Area/LConn1 -- Empirical Factor/RConn1
  mdot_w/RConn1 -- Water Surface Area/RConn1
  Vdot/RConn1 -- Flow Area/LConn1

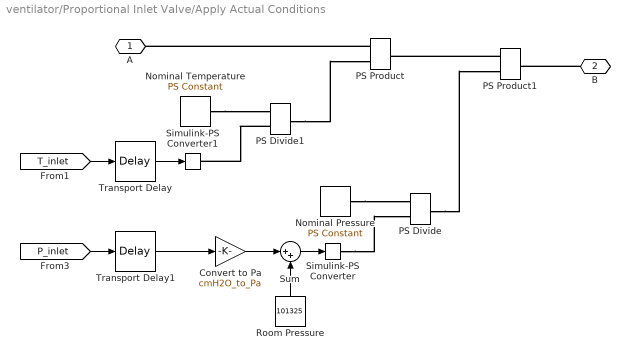
== system ventilator/Proportional Inlet Valve/Apply Actual Conditions ==
  Convert to Pa : Gain  Gain=cmH2O_to_Pa
  Nominal Pressure : fl_lib/Physical Signals/Sources/PS Constant  constant=101325 Pa
  Nominal Temperature : fl_lib/Physical Signals/Sources/PS Constant  constant=273.15+20 K
  PS Divide : fl_lib/Physical Signals/Functions/PS Divide
      settings: SourceProductBaseCode=SS
  PS Divide1 : fl_lib/Physical Signals/Functions/PS Divide
      settings: SourceProductBaseCode=SS
  PS Product : fl_lib/Physical Signals/Functions/PS Product
  PS Product1 : fl_lib/Physical Signals/Functions/PS Product
  Room Pressure : Constant  Value=101325
  Simulink-PS Converter : nesl_utility/Simulink-PS Converter  PhysicalDomain=network_engine_domain  SubClassName=ps_input  LeftPortType=input  RightPortType=output  PseudoPeriodic=off  Frequencies=[]  NoiseDistribution=none  NoiseParameters=[]  Unit=Pa  AffineConversion=off  FilteringAndDerivatives=provide  SimscapeFilterOrder=1  InputFilterTimeConstant=0.001  UdotUserProvided=0
  Simulink-PS Converter1 : nesl_utility/Simulink-PS Converter  PhysicalDomain=network_engine_domain  SubClassName=ps_input  LeftPortType=input  RightPortType=output  PseudoPeriodic=off  Frequencies=[]  NoiseDistribution=none  NoiseParameters=[]  Unit=K  AffineConversion=off  FilteringAndDerivatives=provide  SimscapeFilterOrder=1  InputFilterTimeConstant=0.001  UdotUserProvided=0
  Sum : Sum  Inputs=|++
  Transport Delay : TransportDelay  DelayTime=Transport_Delay  InitialOutput=273.15+T_room  BufferSize=2048
  Transport Delay1 : TransportDelay  DelayTime=Transport_Delay  BufferSize=2048
  A : PMIOPort  Side=Left
  B : PMIOPort  Port=2  Side=Right
  wires:
  [P_inlet] -> Transport Delay1/1
  [T_inlet] -> Transport Delay/1
  Room Pressure/1 -> Sum/2
  Sum/1 -> Simulink-PS Converter/1
  Convert to Pa/1 -> Sum/1
  Transport Delay/1 -> Simulink-PS Converter1/1
  Transport Delay1/1 -> Convert to Pa/1
  connections:
  PS Product/LConn1 -- A/RConn1
  Simulink-PS Converter/RConn1 -- PS Divide/LConn2
  Nominal Pressure/RConn1 -- PS Divide/LConn1
  Nominal Temperature/RConn1 -- PS Divide1/LConn1
  PS Product1/LConn1 -- PS Product/RConn1
  B/RConn1 -- PS Product1/RConn1
  PS Divide1/RConn1 -- PS Product/LConn2
  PS Divide/RConn1 -- PS Product1/LConn2
  PS Divide1/LConn2 -- Simulink-PS Converter1/RConn1

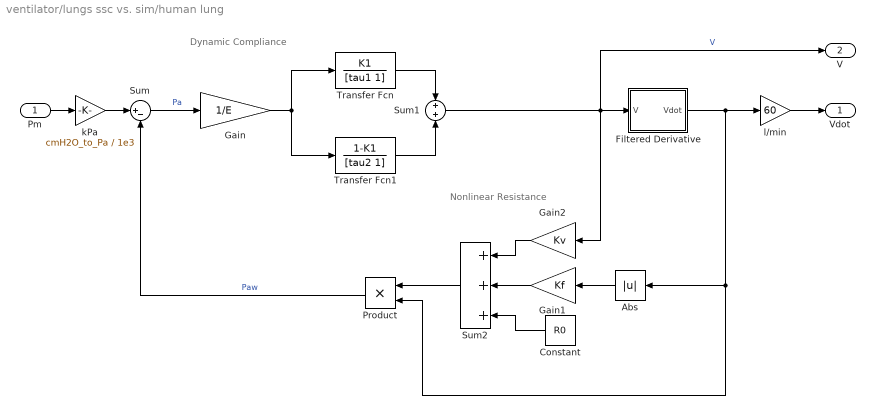
== system ventilator/lungs ssc vs. sim/human lung ==
  note: Nonlinear Resistance
  note: Dynamic Compliance
  Pm : Inport
  Abs : Abs
  Constant : Constant  Value=R0
  Filtered Derivative : Subsystem  mask{sw=on, tau=0.01}
      mask prompts: sw "Enable Filtered Derivative"; tau "Filter time constant [s]"
      mask init:
      | h = find_system(gcb, 'LookUnderMasks', 'all', 'Name', 'Switch');
      | set_param(h{1}, 'sw', num2str(sw));
      mask Callback sw:
      | sw = get_param(gcb, 'sw');
      | if strcmp(sw, 'on')
      |     set_param(gcb, 'MaskEnableString', 'on,on');
      | else
      |     set_param(gcb, 'MaskEnableString', 'on,off');
      | end
      mask Display: disp('du/dt', 'texmode','on');
  Gain : Gain  Gain=1/E
  Gain1 : Gain  Gain=Kf
  Gain2 : Gain  Gain=Kv
  Product : Product
  Sum : Sum  Inputs=|+-
  Sum1 : Sum
  Sum2 : Sum  Inputs=3
  Transfer Fcn : TransferFcn  Numerator=K1  Denominator=[tau1 1]
  Transfer Fcn1 : TransferFcn  Numerator=1-K1  Denominator=[tau2 1]
  kPa : Gain  Gain=cmH2O_to_Pa / 1e3
  l/min : Gain  Gain=60
  Vdot : Outport
  V : Outport  Port=2
  wires:
  Gain/1 -> Transfer Fcn1/1, Transfer Fcn/1
  Sum/1 -> Gain/1  "Pa"
  Transfer Fcn1/1 -> Sum1/2
  Sum1/1 -> Filtered Derivative/1(V), V/1, Gain2/1  "V"
  Pm/1 -> kPa/1
  Abs/1 -> Gain1/1
  Gain2/1 -> Sum2/1
  Gain1/1 -> Sum2/2
  Constant/1 -> Sum2/3
  Product/1 -> Sum/2  "Paw"
  Sum2/1 -> Product/1
  Filtered Derivative/1(Vdot) -> l/min/1, Abs/1, Product/2
  kPa/1 -> Sum/1
  l/min/1 -> Vdot/1
  Transfer Fcn/1 -> Sum1/1

== system ventilator/lungs ssc vs. sim/human lung/Filtered Derivative ==
  V : Inport
  Derivative : Derivative
  Filtered Derivative : TransferFcn  Numerator=[1 0]  Denominator=[tau 1]
  Switch : ManualSwitch
  Vdot : Outport
  wires:
  Switch/1 -> Vdot/1
  Derivative/1 -> Switch/2
  V/1 -> Derivative/1, Filtered Derivative/1
  Filtered Derivative/1 -> Switch/1
